simulink model "TestModel"  (R2023b)
settings: Solver=ode45  StartTime=0.0  StopTime=1  FixedStep=0.0104  RelTol=1e-3
InitFcn:
  | Init_TestModel;
StartFcn:
  | Init_TestModel;
undefined symbols (not defined in the file or in its folder): Norm
libraries: slident x1
settings Model: Creator=Selim  LastModifiedBy=Selim

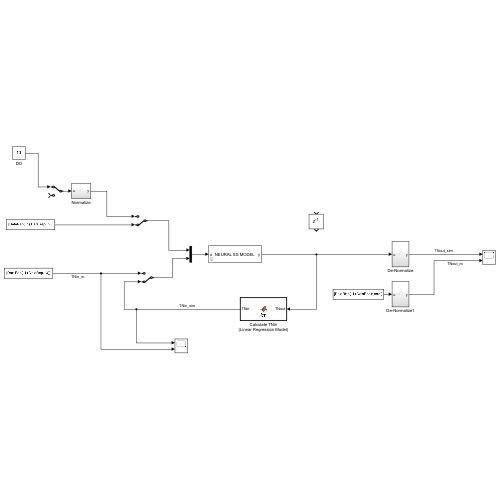
[thumbnail: Simulink's stored preview of the top-level diagram]
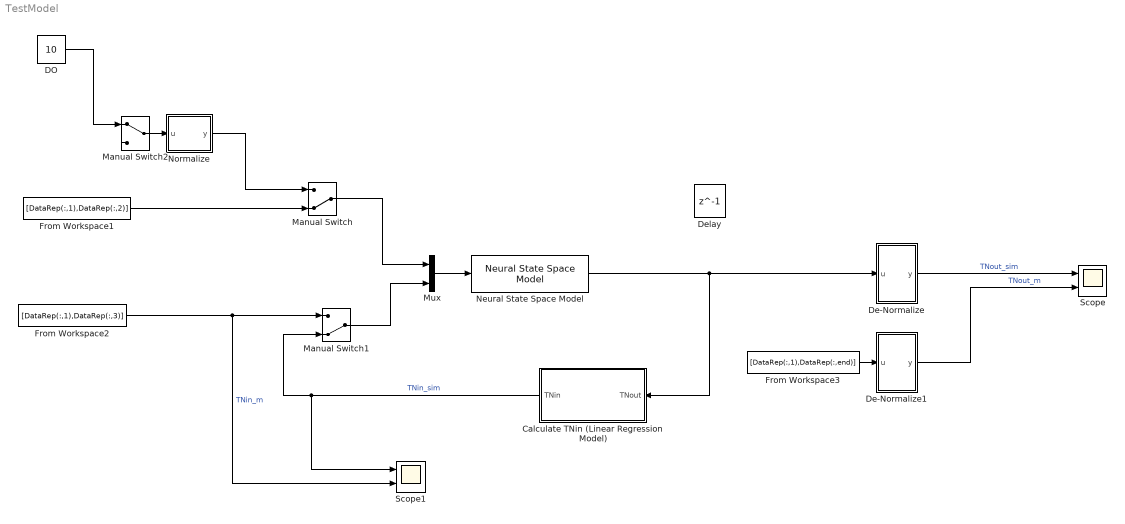
== system TestModel ==
  "Calculate TNin (Linear Regression Model) " : MATLAB Function  TreatAsAtomicUnit=on
  DO : Constant  Value=10
  De-Normalize : Subsystem
  De-Normalize1 : Subsystem
  Delay : Delay  DelayLength=1
  From Workspace1 : FromWorkspace  VariableName=[DataRep(:,1),DataRep(:,2)]
  From Workspace2 : FromWorkspace  VariableName=[DataRep(:,1),DataRep(:,3)]
  From Workspace3 : FromWorkspace  VariableName=[DataRep(:,1),DataRep(:,end)]
  Manual Switch : ManualSwitch  CurrentSetting=0
  Manual Switch1 : ManualSwitch  CurrentSetting=0
  Manual Switch2 : ManualSwitch
  Mux : Mux  Inputs=2
  Neural State Space Model : slident/Models/Neural State Space Model  sys=sys  x0type=internal  ic=0  returnx=off  returndx=off  domain=CT  feedthroughCT=NoFT  feedthroughDT=FT
  Normalize : Subsystem
  Scope : Scope  NumInputPorts=2
  Scope1 : Scope  NumInputPorts=2
  wires:
  Mux/1 -> Neural State Space Model/1
  "Calculate TNin (Linear Regression Model) "/1(TNin) -> Scope1/1, Manual Switch1/2  "TNin_sim"
  Neural State Space Model/1 -> "Calculate TNin (Linear Regression Model) "/1(TNout), De-Normalize/1(u)
  Manual Switch/1 -> Mux/1
  DO/1 -> Manual Switch2/1
  Normalize/1(y) -> Manual Switch/1
  Manual Switch1/1 -> Mux/2
  Manual Switch2/1 -> Normalize/1(u)
  From Workspace1/1 -> Manual Switch/2
  From Workspace2/1 -> Scope1/2, Manual Switch1/1  "TNin_m"
  De-Normalize/1(y) -> Scope/1  "TNout_sim"
  From Workspace3/1 -> De-Normalize1/1(u)
  De-Normalize1/1(y) -> Scope/2  "TNout_m"

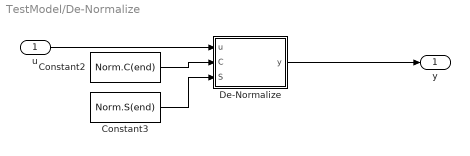
== system TestModel/De-Normalize ==
  u : Inport
  Constant2 : Constant  Value=Norm.C(end)
  Constant3 : Constant  Value=Norm.S(end)
  De-Normalize : MATLAB Function  TreatAsAtomicUnit=on
  y : Outport
  wires:
  Constant2/1 -> De-Normalize/2(C)
  De-Normalize/1(y) -> y/1
  u/1 -> De-Normalize/1(u)
  Constant3/1 -> De-Normalize/3(S)

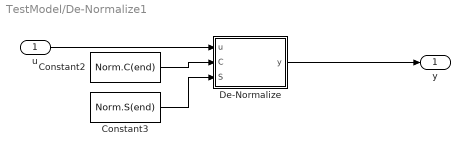
== system TestModel/De-Normalize1 ==
  u : Inport
  Constant2 : Constant  Value=Norm.C(end)
  Constant3 : Constant  Value=Norm.S(end)
  De-Normalize : MATLAB Function  TreatAsAtomicUnit=on
  y : Outport
  wires:
  Constant3/1 -> De-Normalize/3(S)
  u/1 -> De-Normalize/1(u)
  De-Normalize/1(y) -> y/1
  Constant2/1 -> De-Normalize/2(C)

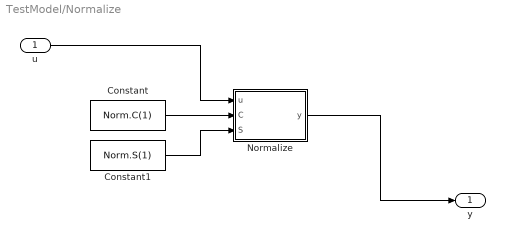
== system TestModel/Normalize ==
  u : Inport
  Constant : Constant  Value=Norm.C(1)
  Constant1 : Constant  Value=Norm.S(1)
  Normalize : MATLAB Function  TreatAsAtomicUnit=on
  y : Outport
  wires:
  u/1 -> Normalize/1(u)
  Constant1/1 -> Normalize/3(S)
  Constant/1 -> Normalize/2(C)
  Normalize/1(y) -> y/1

== matlab function TestModel/Normalize/Normalize ==
  data: u input; y output; C input; S input
function y = fcn(u,C,S)

y = (u - C)/S;

end

== matlab function TestModel/Calculate TNin (Linear Regression Model)  ==
  data: TNout input; TNin output; p_reg parameter
function TNin = fcn(TNout,p_reg)

TNin = polyval(p_reg,TNout);

end

== matlab function TestModel/De-Normalize/De-Normalize ==
  data: u input; y output; C input; S input
function y = fcn(u,C,S)

y = u * S + C;

end

== matlab function TestModel/De-Normalize1/De-Normalize ==
  data: u input; y output; C input; S input
function y = fcn(u,C,S)

y = u * S + C;

end
